simulink model "Fan"  (R2025a)
settings: Solver=VariableStepAuto  StartTime=0.0  StopTime=10.0  RelTol=1e-3
undefined symbols (not defined in the file or in its folder): BPR_design, Eff_Fan_v1, Fan_eta_data, Fan_PR_data, flow_vec_fan, speed_vec_fan
settings Model: Creator=ramch  LastModifiedBy=ramch

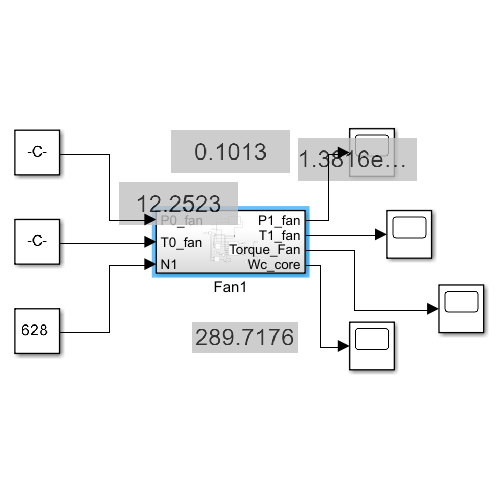
[thumbnail: Simulink's stored preview of the top-level diagram]
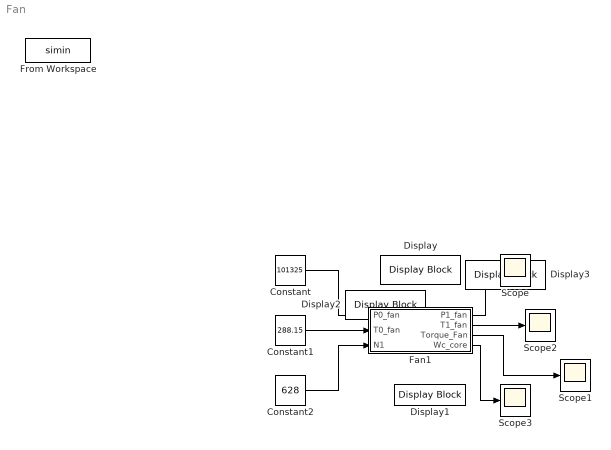
== system Fan ==
  Constant : Constant  Value=101325
  Constant1 : Constant  Value=288.15
  Constant2 : Constant  Value=628
  Display{,1..3} (4 alike) : DisplayBlock  LabelPosition=Hide  Transparency=1  GridColor=[0.502, 0.502, 0.502]
  Fan1 : Subsystem
  Scope{,1..3} (4 alike) : Scope
      Scope settings: ActiveDisplayYMinimum=-1  ActiveDisplayYMaximum=1
      Scope1 settings: ActiveDisplayYMinimum=-1  ActiveDisplayYMaximum=1
      Scope2 settings: ActiveDisplayYMinimum=-1  ActiveDisplayYMaximum=1  DataLoggingVariableName=ScopeData2
      Scope3 settings: ActiveDisplayYMinimum=-1  ActiveDisplayYMaximum=1  DataLoggingVariableName=ScopeData3
  From Workspace : FromWorkspace  IOType=siggen  VariableName=simin  ZeroCross=off
  wires:
  Fan1/4(Wc_core) -> Scope3/1
  Fan1/3(Torque_Fan) -> Scope1/1
  Fan1/2(T1_fan) -> Scope2/1
  Fan1/1(" P1_fan") -> Scope/1
  Constant2/1 -> Fan1/3(N1)
  Constant1/1 -> Fan1/2(T0_fan)
  Constant/1 -> Fan1/1(P0_fan)

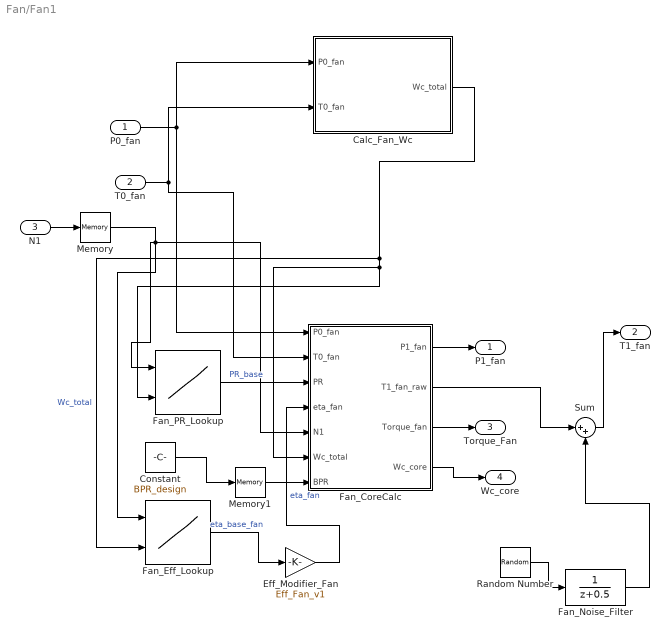
== system Fan/Fan1 ==
  P0_fan : Inport
  T0_fan : Inport  Port=2
  N1 : Inport  Port=3
  Calc_Fan_Wc : MATLAB Function  TreatAsAtomicUnit=on
  Constant : Constant  Value=BPR_design
  Eff_Modifier_Fan : Gain  Gain=Eff_Fan_v1
  Fan_CoreCalc : MATLAB Function  TreatAsAtomicUnit=on
  Fan_Eff_Lookup : Lookup_n-D  BreakpointsForDimension1=speed_vec_fan  BreakpointsForDimension2=flow_vec_fan  Table=Fan_eta_data  InternalRulePriority=Speed  RndMeth=Simplest
      settings: InputPortMap=u0,u1
  Fan_Noise_Filter : DiscreteTransferFcn
  Fan_PR_Lookup : Lookup_n-D  BreakpointsForDimension1=speed_vec_fan  BreakpointsForDimension2=flow_vec_fan  Table=Fan_PR_data  InternalRulePriority=Speed  RndMeth=Simplest
      settings: InputPortMap=u0,u1
  Memory : Memory
  Memory1 : Memory
  Random Number : RandomNumber  Variance=(0.5)  SampleTime=0.001
  Sum : Sum  Inputs=|++
  " P1_fan" : Outport
  T1_fan : Outport  Port=2
  Torque_Fan : Outport  Port=3
  Wc_core : Outport  Port=4
  wires:
  Random Number/1 -> Fan_Noise_Filter/1
  Fan_Noise_Filter/1 -> Sum/2
  Fan_CoreCalc/2(T1_fan_raw) -> Sum/1
  Sum/1 -> T1_fan/1
  Fan_CoreCalc/1(P1_fan) -> " P1_fan"/1
  Fan_CoreCalc/3(Torque_fan) -> Torque_Fan/1
  Fan_CoreCalc/4(Wc_core) -> Wc_core/1
  Fan_PR_Lookup/1 -> Fan_CoreCalc/3(PR)  "PR_base"
  Eff_Modifier_Fan/1 -> Fan_CoreCalc/4(eta_fan)  "eta_fan"
  Fan_Eff_Lookup/1 -> Eff_Modifier_Fan/1  "eta_base_fan"
  Calc_Fan_Wc/1(Wc_total) -> Fan_Eff_Lookup/2, Fan_PR_Lookup/2, Fan_CoreCalc/6(Wc_total)  "Wc_total"
  T0_fan/1 -> Calc_Fan_Wc/2(T0_fan), Fan_CoreCalc/2(T0_fan)
  P0_fan/1 -> Calc_Fan_Wc/1(P0_fan), Fan_CoreCalc/1(P0_fan)
  Memory1/1 -> Fan_CoreCalc/7(BPR)
  Memory/1 -> Fan_PR_Lookup/1, Fan_CoreCalc/5(N1), Fan_Eff_Lookup/1
  N1/1 -> Memory/1
  Constant/1 -> Memory1/1

== matlab function Fan/Fan1/Calc_Fan_Wc ==
  data: P0_fan input; Wc_total output; T0_fan input
function Wc_total = Calc_Fan_Wc(P0_fan, T0_fan)
% Computes corrected total mass flow (core+bypass) [kg/s]

    % Constants
    Tref = 288.15;       % [K]
    Pref = 101325;       % [Pa]
    R = 287;             % [J/(kg·K)]
    A = 0.50;            % [m^2], approximated fan face area
    V = 120;             % [m/s], estimated inlet velocity

    % Density at inlet
    rho = P0_fan / (R * T0_fan);

    % Actual total mass flow
    m_dot_total = rho * A * V;  % [kg/s]

    % Corrected mass flow
    Wc_total = m_dot_total / sqrt(T0_fan / Tref) * (Pref / P0_fan);
end

== matlab function Fan/Fan1/Fan_CoreCalc ==
  data: P0_fan input; P1_fan output; T0_fan input; PR input; eta_fan input; N1 input; Wc_total input; BPR input; T1_fan_raw output; Torque_fan output; Wc_core output
function [P1_fan, T1_fan_raw, Torque_fan, Wc_core] = Fan_CoreCalc(...
          P0_fan, T0_fan, PR, eta_fan, N1, Wc_total, BPR)
% Fan thermodynamics and torque

    gamma = 1.4;
    cp = 1004;  % J/(kg·K)
    % 1) Outlet total pressure
    PR = max(PR, 1e-6);  % prevent PR ≤ 0
    P1_fan = max(P0_fan .* PR, 1e-6);    
    % 2) Outlet total temperature (isentropic + efficiency)
    T1_fan_raw = T0_fan * (1 + (1/eta_fan) * (PR^((gamma-1)/gamma) - 1));
    % 3) Convert N1 (RPM) to rad/s
    omega1 = max(N1 * 2 * pi / 60, eps); % eps = tiny nonzero value;
    % 4) Recover actual mass flow from Wc_total
    Tref = 288.15; Pref = 101325;
    m_dot_total = Wc_total * sqrt(T0_fan / Tref) * (P0_fan / Pref);
    % 5) Split flow: core vs bypass
    m_dot_core = m_dot_total / (1 + BPR);
    % 6) Core corrected flow for downstream: 
    Wc_core = m_dot_core / sqrt(T0_fan / Tref) * (Pref / P0_fan);
    % 7) Enthalpy rise
    delta_h = cp * (T1_fan_raw - T0_fan);
    % 8) Torque on shaft
    Torque_fan = (m_dot_total * delta_h) / omega1;
end
